simulink model "Tricopter"  (R2016b)
settings: Solver=VariableStepAuto  StartTime=0.0  StopTime=10.0  RelTol=1e-3
values from neighbouring files (symbols this model uses):
  g = 9.81    [main.m]
  I = [0.00025 0 2.55e-6; 0 0.000232 0; 2.55e-6 0 0.0003738]    [main.m]
  kf = 6.11*10^-8    (= 6.11e-08)    [main.m]
  km = 1.5*10^-9    (= 1.5e-09)    [main.m]
  m = 0.18    [main.m]
undefined symbols (not defined in the file or in its folder): invI, L
libraries: vrlib x1, dspmtrx3 x1
settings Model: Creator=Nu  LastModifiedBy=Nu

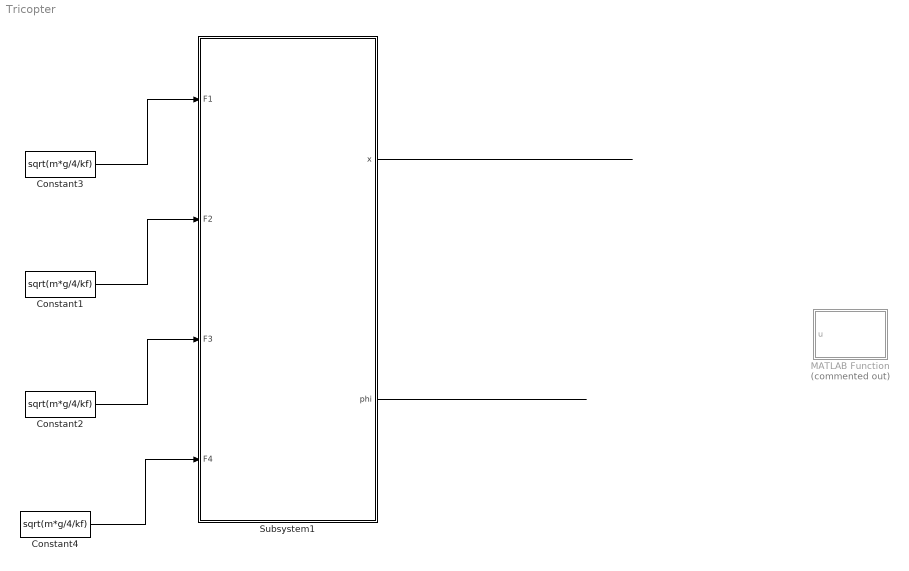
== system Tricopter ==
  Constant{1..4} (4 alike) : Constant  Value=sqrt(m*g/4/kf)
  MATLAB Function : MATLAB Function  Commented=on  TreatAsAtomicUnit=on
  Subsystem1 : Subsystem
  wires:
  Constant2/1 -> Subsystem1/3(F3)
  Constant1/1 -> Subsystem1/2(F2)
  Constant3/1 -> Subsystem1/1(F1)
  Constant4/1 -> Subsystem1/4(F4)
  Subsystem1/1(x) -> ?
  Subsystem1/2(phi) -> ?

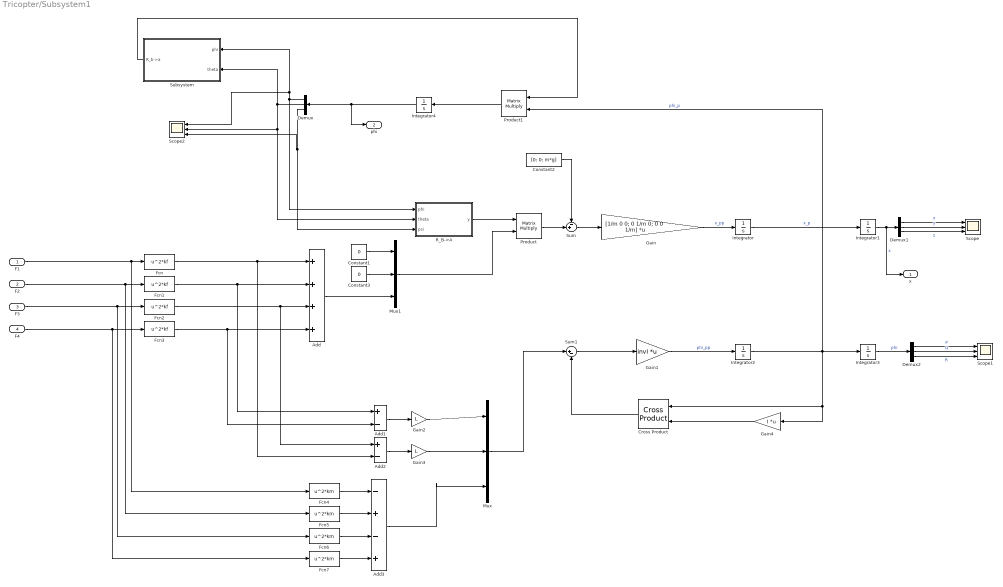
== system Tricopter/Subsystem1 ==
  F1 : Inport
  F2 : Inport  Port=2
  F3 : Inport  Port=3
  F4 : Inport  Port=4
  Add : Sum  Inputs=++++
  Add1 : Sum  Inputs=+-
  Add2 : Sum  Inputs=+-
  Add3 : Sum  Inputs=-+-+
  Constant1 : Constant  Value=0
  Constant2 : Constant  Value=[0; 0; m*g]
  Constant3 : Constant  Value=0
  Cross Product : vrlib/Utilities/Cross Product
  Demux : Demux  Outputs=3
  Demux1 : Demux  Outputs=3
  Demux2 : Demux  Outputs=3
  Fcn{,1..3} (4 alike) : Fcn  Expr=u^2*kf
  Fcn{4..7} (4 alike) : Fcn  Expr=u^2*km
  Gain : Gain  Gain=[1/m 0 0; 0 1/m 0; 0 0 1/m]  Multiplication=Matrix(K*u)
  Gain1 : Gain  Gain=invI  Multiplication=Matrix(K*u)
  Gain2 : Gain  Gain=L
  Gain3 : Gain  Gain=L
  Gain4 : Gain  Gain=I  Multiplication=Matrix(K*u)
  Integrator{,1..4} (5 alike) : Integrator
  Mux : Mux  Inputs=3
  Mux1 : Mux  Inputs=3
  Product : Product  Multiplication=Matrix(*)
  Product1 : Product  Multiplication=Matrix(*)
  R_B->A : MATLAB Function  TreatAsAtomicUnit=on
  Scope : Scope  NumInputPorts=3
  Scope1 : Scope  NumInputPorts=3
  Scope2 : Scope  NumInputPorts=3
  Subsystem : Subsystem
  Sum : Sum  Inputs=-+|
  Sum1 : Sum  Inputs=|+-
  x : Outport
  phi : Outport  Port=2
  wires:
  R_B->A/1(y) -> Product/1
  Subsystem/1(R_b->a) -> Product1/1
  Constant2/1 -> Sum/1
  Add/1 -> Mux1/3
  Product/1 -> Sum/2
  Sum/1 -> Gain/1
  Gain/1 -> Integrator/1  "x_pp"
  Integrator/1 -> Integrator1/1  "x_p"
  Integrator1/1 -> x/1, Demux1/1  "x"
  Integrator2/1 -> Integrator3/1, Gain4/1, Cross Product/1, Product1/2  "phi_p"
  Demux/1 -> Scope2/1, Subsystem/1(phi), R_B->A/1(phi)
  Gain1/1 -> Integrator2/1  "phi_pp"
  Integrator3/1 -> Demux2/1  "phi"
  Demux/2 -> Subsystem/2(theta), Scope2/2, R_B->A/2(theta)
  Demux/3 -> Scope2/3, R_B->A/3(psi)
  Integrator4/1 -> phi/1, Demux/1
  Product1/1 -> Integrator4/1
  F2/1 -> Fcn5/1, Fcn1/1
  F4/1 -> Fcn7/1, Fcn3/1
  F3/1 -> Fcn6/1, Fcn2/1
  F1/1 -> Fcn4/1, Fcn/1
  Add1/1 -> Gain2/1
  Add2/1 -> Gain3/1
  Add3/1 -> Mux/3
  Gain2/1 -> Mux/1
  Gain3/1 -> Mux/2
  Mux/1 -> Sum1/1
  Sum1/1 -> Gain1/1
  Gain4/1 -> Cross Product/2
  Cross Product/1 -> Sum1/2
  Constant1/1 -> Mux1/1
  Mux1/1 -> Product/2
  Constant3/1 -> Mux1/2
  Demux1/1 -> Scope/1  "x"
  Demux1/2 -> Scope/2  "y"
  Demux1/3 -> Scope/3  "z"
  Demux2/1 -> Scope1/1  "P"
  Demux2/2 -> Scope1/2  "Q"
  Demux2/3 -> Scope1/3  "R"
  Fcn/1 -> Add2/2, Add/1
  Fcn1/1 -> Add1/1, Add/2
  Fcn2/1 -> Add2/1, Add/3
  Fcn3/1 -> Add1/2, Add/4
  Fcn4/1 -> Add3/1
  Fcn5/1 -> Add3/2
  Fcn7/1 -> Add3/4
  Fcn6/1 -> Add3/3

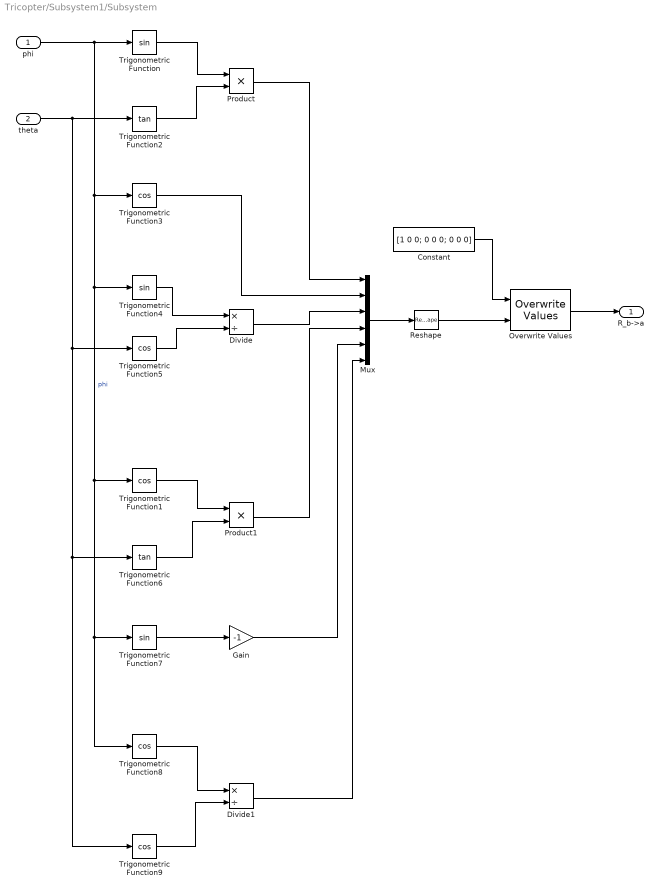
== system Tricopter/Subsystem1/Subsystem ==
  phi : Inport
  theta : Inport  Port=2
  Constant : Constant  Value=[1 0 0; 0 0 0; 0 0 0]
  Divide : Product  Inputs=*/
  Divide1 : Product  Inputs=*/
  Gain : Gain  Gain=-1
  Mux : Mux  Inputs=6
  Overwrite Values : dspmtrx3/Overwrite Values  OverWriteDiag=Submatrix  valFrom2ndIP=Second input port  ConstValue=0  RowSpan=Range of rows  RowStartMode=First  RowStartIndex=1  RowEndMode=Last  RowEndIndex=1  ColSpan=Range of columns  ColStartMode=Index  ColStartIndex=2  ColEndMode=Last  ColEndIndex=1  DiagSpan=Range of elements  DiagStartMode=Index  DiagStartIndex=2  DiagEndMode=Index  DiagEndIndex=4
  Product : Product
  Product1 : Product
  Reshape : Reshape  OutputDimensionality=Customize  OutputDimensions=[3,2]
  Trigonometric Function : Trigonometry
  Trigonometric Function{1,3,5,8..9} (5 alike) : Trigonometry  Operator=cos
  Trigonometric Function2 : Trigonometry  Operator=tan
  Trigonometric Function4 : Trigonometry
  Trigonometric Function6 : Trigonometry  Operator=tan
  Trigonometric Function7 : Trigonometry
  R_b->a : Outport
  wires:
  Trigonometric Function1/1 -> Product1/1
  Trigonometric Function2/1 -> Product/2
  Trigonometric Function/1 -> Product/1
  Mux/1 -> Reshape/1
  phi/1 -> Trigonometric Function4/1, Trigonometric Function7/1, Trigonometric Function8/1, Trigonometric Function1/1, Trigonometric Function3/1, Trigonometric Function/1  "phi"
  theta/1 -> Trigonometric Function9/1, Trigonometric Function6/1, Trigonometric Function5/1, Trigonometric Function2/1
  Trigonometric Function5/1 -> Divide/2
  Trigonometric Function4/1 -> Divide/1
  Trigonometric Function3/1 -> Mux/2
  Trigonometric Function6/1 -> Product1/2
  Product/1 -> Mux/1
  Divide/1 -> Mux/3
  Product1/1 -> Mux/4
  Trigonometric Function7/1 -> Gain/1
  Trigonometric Function8/1 -> Divide1/1
  Trigonometric Function9/1 -> Divide1/2
  Gain/1 -> Mux/5
  Divide1/1 -> Mux/6
  Reshape/1 -> Overwrite Values/2
  Constant/1 -> Overwrite Values/1
  Overwrite Values/1 -> R_b->a/1

== matlab function Tricopter/MATLAB Function ==
  data: u input
function fcn(u)

QP.UpdateQuadPlot(x, [desired_state.pos; desired_state.vel], time);

== matlab function Tricopter/Subsystem1/R_B->A ==
  data: phi input; theta input; psi input; y output
function y = fcn(phi, theta, psi)

y = [cos(theta)*cos(psi) sin(theta)*sin(phi)*cos(psi)+cos(phi)*sin(psi) sin(theta)*cos(phi)*cos(psi)-sin(phi)*sin(psi); ...
     cos(theta)*sin(psi) sin(theta)*sin(phi)*sin(psi)-cos(phi)*cos(psi) sin(theta)*cos(phi)*sin(psi)-sin(phi)*cos(psi); ...
     -sin(theta)        cos(theta)*sin(psi)    cos(theta)*cos(phi)];
